simulink model "sfcndemo_lqry"  (Simulink 7.1)
settings: Solver=FixedStepDiscrete  StartTime=0.0  StopTime=10  FixedStep=.01  RelTol=1e-3
InitFcn:
  | al   = 1;
  | be   = 1;
  | th   = .03/1000;
  | w    = .011;
  | rR   = .01;
  | rS   = .01;
  | rW   = .01;
  | vR = .001;
  | vS = .001;
  | vW = .001;
  | A   =   [  0 0 0 1 0 0;
  |               0 0 0 0 1 0;
  |               0 0 0 0 0 1;
  |               3*w^2 0 0 0 2*w 0;
  |               0 0 0 -2*w 0 0;
  |               0 0 -w^2 0 0 0];
  | B   =   [  zeros(3);eye(3)];
  | Q   =  diag([al^2/rR^2,al^2/rS^2,al^2/rW^2,al^2/vR^2,al^2/vS^2,al^2/vW^2]);
  | R   =  diag([be^2/th^2,be^2/th^2,be^2/th^2]);
  | [n,m] = size(B);
  | p = size(Q,1);
  | C = eye(p);
  | D = zeros(p,m);
  | 
  | %[K,S,E] = lqry(A,B,C,D,Q,R)
settings Model: Creator=Administrator  LastModifiedBy=campa  ExtModeAutoUpdateStatusClock=off
settings DataIOCC: LimitDataPoints=off  SaveOutput=off  SaveTime=off
settings OptimizationCC: BlockReduction=off  BooleanDataType=off
settings DebuggingCC: SaveWithParameterizedLinksMsg=none  SignalResolutionControl=TryResolveAllWithWarning  SolverPrmCheckMsg=none  MultiTaskDSMMsg=warning  MultiTaskCondExecSysMsg=none  StrictBusMsg=None
settings RTWCC: RTWVerbose=off  ProcessScript=grt_make_rtw_hook  CustomInclude=src  IncludeERTFirstTime=on
settings RTWCC: CustomSource=|
  | balgbk.o d1nrm.o dgefam.o drot.o dswap.o gradbk.o lineq.o mlineq.o mqfwo.o mulb.o
  | orthes.o qzval.o rinv.o scalbk.o symslv.o balgen.o daxpy.o dgeslm.o dscal.o exchqz.o
  | gradeq.o lypcnd.o mmul.o mscale.o mulwoa.o ortran.o reduce.o rotc.o scaleg.o trnata.o
  | cmprs.o ddot.o dnrm2.o dstslv.o fbgain.o hqrort.o lypdsd.o mqfa.o msub.o newt.o qzhesw.o
  | resid.o rotr.o sepest.o trnatb.o creg.o dgecom.o drotg.o dsvdc.o giv.o madd.o mqf.o
  | mula.o order.o qzitw.o ricsol.o save.o symprd.o xty.o

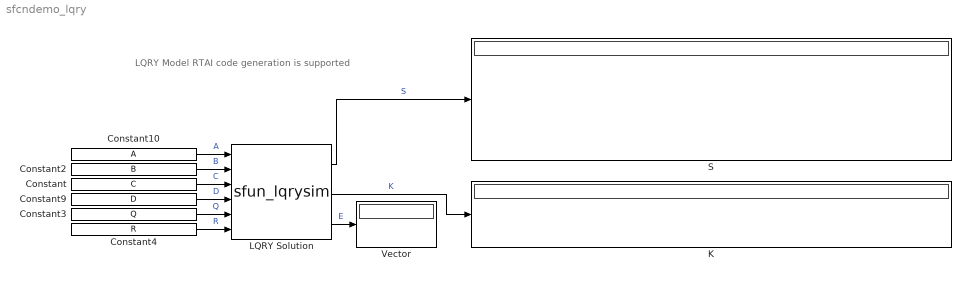
== system sfcndemo_lqry ==
  note: LQRY Model
      | RTAI code generation is supported
  " Vector " : Display
  Constant : Constant  Value=C  VectorParams1D=off
  Constant10 : Constant  Value=A  VectorParams1D=off
  Constant2 : Constant  Value=B  VectorParams1D=off
  Constant3 : Constant  Value=Q  VectorParams1D=off
  Constant4 : Constant  Value=R  VectorParams1D=off
  Constant9 : Constant  Value=D  VectorParams1D=off
  K : Display
  LQRY Solution : S-Function  FunctionName=sfun_lqrysim  Parameters=n, m, p  EnableBusSupport=off  mask(LQRY Linear-quadratic regulator design with output weighting (for Simulink)){n=6, m=3, p=6}
      mask prompts: n "Enter the Number of States:"; m "Enter the Number of Controls:"; p "Enter the Number of Outputs:"
      mask help:
      | This block calculates the optimal gain matrix K such that
      | the state-feedback law u = -Kx  minimizes the cost function:
      |               J = Integral {y'Qy + u'Ru} dt                                    .
      |  subject to the system dynamics  x = Ax + Bu,  y = Cx + Du
      | Inputs to the block are A, B, C, D, Q and R in matrix form.  Also, the
      | number of states, number of controls and number of outputs are required as
      | parameters to the mask.  Returned are the solution S in matrix form of the
      | associated algebraic Riccati equation and a 2D vector.  The first element
      | in the 2D vector indicates an error when greater than zero or a somewhat
      | "unreliable" result when negative.  The second element is the condition
      | number of the R matrix.
      mask Display:
      | disp('LQRY')
      | 
      | port_label('input',1,'\bfA','texmode','on')
      | port_label('input',2,'\bfB','texmode','on')
      | port_label('input',3,'\bfC','texmode','on')
      | port_label('input',4,'\bfD','texmode','on')
      | port_label('input',5,'\bfQ','texmode','on')
      | port_label('input',6,'\bfR','texmode','on')
      | 
      | port_label('output',1,'\bfS','texmode','on')
      | port_label('output',2,'\bfK','texmode','on')
      | port_label('output',3,'\bfE','texmode','on')
  S : Display
  wires:
  LQRY Solution/1 -> S/1  "S"
  LQRY Solution/2 -> K/1  "K"
  LQRY Solution/3 -> " Vector "/1  "E"
  Constant10/1 -> LQRY Solution/1  "A"
  Constant2/1 -> LQRY Solution/2  "B"
  Constant/1 -> LQRY Solution/3  "C"
  Constant9/1 -> LQRY Solution/4  "D"
  Constant3/1 -> LQRY Solution/5  "Q"
  Constant4/1 -> LQRY Solution/6  "R"
